simulink model "RCAM_simulation_MIMO"  (R2021b)
settings: Solver=VariableStepAuto  StartTime=0.0  StopTime=TF  FixedStep=0.0001  RelTol=1e-3
values from neighbouring files (symbols this model uses):
  h0 = 1000    [initializeConstantsMIMO.m]
  k = k_gain.K    [initializeConstantsMIMO.m]
  lat0 = convert_coordinates(21, 18, 56.1708)    [initializeConstantsMIMO.m]
  lon0 = convert_coordinates(157, 51, 29.1348)    [initializeConstantsMIMO.m]
  u1max = 25*pi/180    (= 0.436332312999)    [initializeConstantsMIMO.m]
  u1min = -25*pi/180    (= -0.436332312999)    [initializeConstantsMIMO.m]
  u2max = 10*pi/180    (= 0.174532925199)    [initializeConstantsMIMO.m]
  u2min = -25*pi/180    (= -0.436332312999)    [initializeConstantsMIMO.m]
  u3max = 30*pi/180    (= 0.523598775598)    [initializeConstantsMIMO.m]
  u3min = -30*pi/180    (= -0.523598775598)    [initializeConstantsMIMO.m]
  u4max = 1    [initializeConstantsMIMO.m]
  u4min = 0    [initializeConstantsMIMO.m]
  uo = [0 ... (first row only)    [initializeConstantsMIMO.m]
  x0 = [14 ... (first row only)    [initializeConstantsMIMO.m]
undefined symbols (not defined in the file or in its folder): RCAM_model
libraries: aerolibfltsims x2, slpidlib x1
settings Model: PacingRate=3  Creator=khanh  LastModifiedBy=khanh

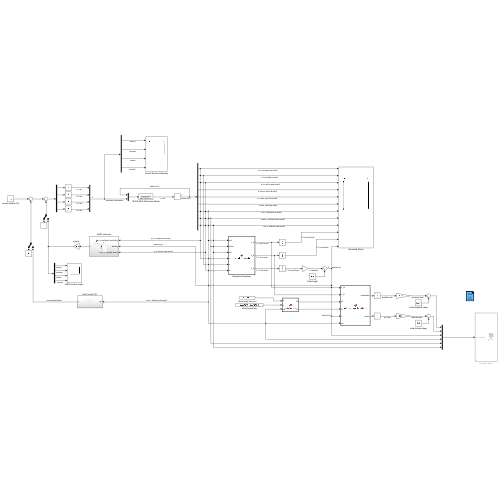
[thumbnail: Simulink's stored preview of the top-level diagram]
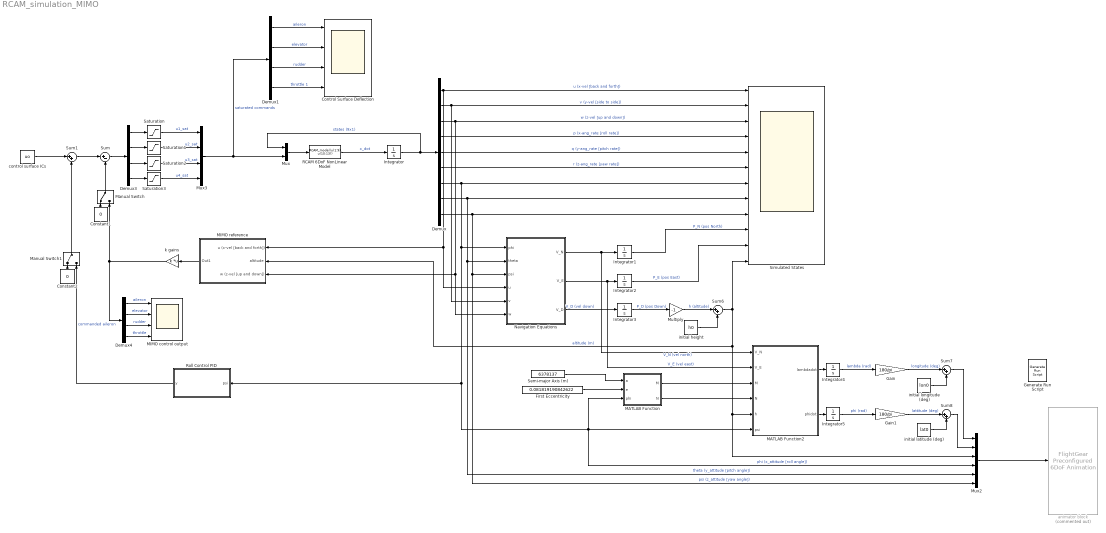
== system RCAM_simulation_MIMO ==
  Constant1 : Constant  Value=0
  Constant2 : Constant  Value=0
  Control Surface Deflection : Scope  NumInputPorts=4
  Demux : Demux  Outputs=9
  Demux1 : Demux
  Demux3 : Demux
  Demux4 : Demux
  First Eccentricity : Constant  Value=0.081819190842622
  Gain : Gain  Gain=180/pi
  Gain1 : Gain  Gain=180/pi
  Generate Run Script : aerolibfltsims/Generate Run Script  Architecture=Win64  dataFlow=Send  GeometryModelName=c172p  AirportId=KSFO  RunwayId=10L  InitialAltitude=7224  InitialHeading=113  OffsetDistance=4.72  OffsetAzimuth=0  InstallScenery=off  DisableShaders=on  OriginAddress=127.0.0.1  DestinationPort=5502  OriginPort=5505  LocalAddress=127.0.0.1  OutputFileName=runfg.bat  FlightGearBaseDirectory=C:\Program Files\FlightGear 2020.3
  Integrator : Integrator  InitialCondition=x0
  Integrator{1..4} (4 alike) : Integrator
  Integrator5 : Integrator  UpperSaturationLimit=pi  LowerSaturationLimit=-pi
  MATLAB Function : MATLAB Function  TreatAsAtomicUnit=on
  MATLAB Function2 : MATLAB Function  TreatAsAtomicUnit=on
  MIMO control output : Scope  NumInputPorts=4
  MIMO reference : Subsystem
  Manual Switch : ManualSwitch
  Manual Switch1 : ManualSwitch
  Multiply : Gain  Gain=-1
  Mux : Mux  Inputs=2
  Mux2 : Mux  Inputs=6
  Mux3 : Mux
  Navigation Equations : MATLAB Function  TreatAsAtomicUnit=on
  RCAM 6DoF NonLinear Model : MATLABFcn  MATLABFcn=RCAM_model(u(1:9), u(10:13))
  Roll Control PID : Subsystem
  Saturation : Saturate  UpperLimit=u1max  LowerLimit=u1min
  Saturation1 : Saturate  UpperLimit=u2max  LowerLimit=u2min
  Saturation2 : Saturate  UpperLimit=u3max  LowerLimit=u3min
  Saturation3 : Saturate  UpperLimit=u4max  LowerLimit=u4min
  Semi-major Axis (m) : Constant  Value=6378137
  Simulated States : Scope  NumInputPorts=12
  Sum : Sum  Inputs=|+-
  Sum{1,6..8} (4 alike) : Sum  Inputs=|++
  animator block : aerolibfltsims/FlightGear Preconfigured 6DoF Animation  Commented=on  xFlightGearVersion=v2019.1  DestinationIpAddress=127.0.0.1  DestinationPort=5502  SampleTime=1/30  packetVersion=24
  control surface ICs : Constant  Value=uo
  initial height : Constant  Value=h0
  initial latitude (deg) : Constant  Value=lat0
  initial longitude (deg) : Constant  Value=lon0
  k gains : Gain  Gain=k  Multiplication=Matrix(K*u)
  wires:
  RCAM 6DoF NonLinear Model/1 -> Integrator/1  "x_dot"
  Mux/1 -> RCAM 6DoF NonLinear Model/1
  Mux3/1 -> Demux1/1, Mux/2  "saturated commands"
  Demux1/1 -> Control Surface Deflection/1  "aileron"
  Demux1/2 -> Control Surface Deflection/2  "elevator"
  Demux1/3 -> Control Surface Deflection/3  "rudder"
  Demux1/4 -> Control Surface Deflection/4  "throttle 1"
  Demux/4 -> Simulated States/4  "p (x-ang_rate [roll rate])"
  Demux/5 -> Simulated States/5  "q (y-ang_rate [pitch rate])"
  Demux/6 -> Simulated States/6  "r (z-ang_rate [yaw rate])"
  Demux/9 -> Mux2/6, Navigation Equations/3(psi), Simulated States/9  "psi (z_attitude [yaw angle])"
  Navigation Equations/3(V_D) -> Integrator3/1  "V_D (vel down)"
  Navigation Equations/2(V_E) -> Integrator2/1, MATLAB Function2/2(V_E)  "V_E (vel east)"
  Navigation Equations/1(V_N) -> MATLAB Function2/1(V_N), Integrator1/1  "V_N (vel north)"
  Integrator1/1 -> Simulated States/10  "P_N (pos North)"
  Integrator2/1 -> Simulated States/11  "P_E (pos East)"
  Integrator3/1 -> Multiply/1  "P_D (pos Down)"
  Semi-major Axis (m)/1 -> MATLAB Function/1(a)
  First Eccentricity/1 -> MATLAB Function/2(e)
  MATLAB Function/2(N) -> MATLAB Function2/4(N)
  MATLAB Function/1(M) -> MATLAB Function2/3(M)
  Demux/7 -> Roll Control PID/1(psi), MATLAB Function2/6(psi), MATLAB Function/3(phi), Mux2/4, Navigation Equations/1(phi), Simulated States/7  "phi (x_attitude [roll angle])"
  Integrator5/1 -> Gain1/1  "phi (rad)"
  Integrator4/1 -> Gain/1  "lambda (rad)"
  Gain/1 -> Sum7/1  "longitude (deg)"
  Multiply/1 -> Sum6/1  "h (altitude)"
  Sum6/1 -> Simulated States/12, MIMO reference/2(altitude), Mux2/3, MATLAB Function2/5(h)  "altitude (m)"
  initial height/1 -> Sum6/2
  MATLAB Function2/1(lambdadot) -> Integrator4/1
  MATLAB Function2/2(phidot) -> Integrator5/1
  Gain1/1 -> Sum8/1  "lattitude (deg)"
  initial longitude (deg)/1 -> Sum7/2
  initial latitude (deg)/1 -> Sum8/2
  Sum7/1 -> Mux2/1
  Sum8/1 -> Mux2/2
  Roll Control PID/1(y) -> Manual Switch1/2  "commanded aileron"
  Saturation3/1 -> Mux3/4  "u4_sat"
  Saturation/1 -> Mux3/1  "u1_sat"
  Saturation1/1 -> Mux3/2  "u2_sat"
  Saturation2/1 -> Mux3/3  "u3_sat"
  Demux3/1 -> Saturation/1
  Demux3/2 -> Saturation1/1
  Demux3/3 -> Saturation2/1
  Demux3/4 -> Saturation3/1
  Demux/3 -> MIMO reference/3(w (z-vel [up and down])), Navigation Equations/6(w), Simulated States/3  "w (z-vel [up and down])"
  Demux/8 -> Mux2/5, Navigation Equations/2(theta), Simulated States/8  "theta (y_attitude [pitch angle])"
  Demux/1 -> Simulated States/1, Navigation Equations/4(u), MIMO reference/1(u (x-vel [back and forth]))  "u (x-vel [back and forth])"
  Demux/2 -> Simulated States/2, Navigation Equations/5(v)  "v (y-vel [side to side])"
  Sum/1 -> Demux3/1
  k gains/1 -> Manual Switch/2, Demux4/1
  Manual Switch/1 -> Sum/2
  Constant1/1 -> Manual Switch/1
  Constant2/1 -> Manual Switch1/1
  Demux4/3 -> MIMO control output/3  "rudder"
  Demux4/4 -> MIMO control output/4  "throttle"
  Demux4/2 -> MIMO control output/2  "elevator"
  Demux4/1 -> MIMO control output/1  "aileron"
  Integrator/1 -> Mux/1, Demux/1  "states (9x1)"
  Mux2/1 -> animator block/1
  Sum1/1 -> Sum/1
  control surface ICs/1 -> Sum1/1
  MIMO reference/1(Out1) -> k gains/1
  Manual Switch1/1 -> Sum1/2

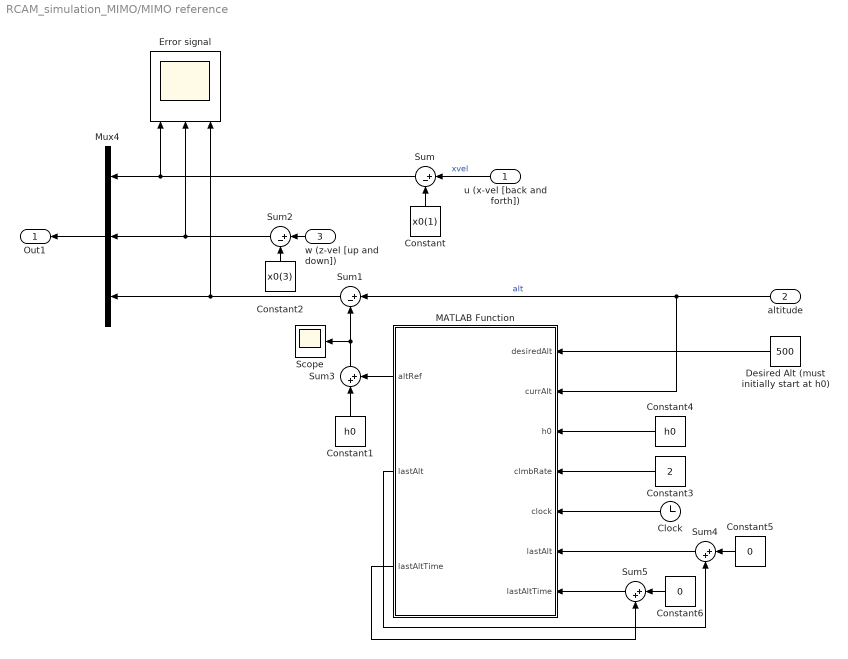
== system RCAM_simulation_MIMO/MIMO reference ==
  u (x-vel [back and forth]) : Inport
  altitude : Inport  Port=2
  w (z-vel [up and down]) : Inport  Port=3
  Clock : Clock
  Constant : Constant  Value=x0(1)
  Constant1 : Constant  Value=h0
  Constant2 : Constant  Value=x0(3)
  Constant3 : Constant  Value=2
  Constant4 : Constant  Value=h0
  Constant5 : Constant  Value=0
  Constant6 : Constant  Value=0
  Desired Alt (must initially start at h0) : Constant  Value=500
  Error signal : Scope  NumInputPorts=3
  MATLAB Function : MATLAB Function  TreatAsAtomicUnit=on
  Mux4 : Mux  Inputs=3
  Scope : Scope
  Sum : Sum  Inputs=|+-
  Sum1 : Sum  Inputs=|+-
  Sum2 : Sum  Inputs=|+-
  Sum3 : Sum  Inputs=|++
  Sum4 : Sum  Inputs=|++
  Sum5 : Sum  Inputs=|++
  Out1 : Outport
  wires:
  Mux4/1 -> Out1/1
  u (x-vel [back and forth])/1 -> Sum/1  "xvel"
  Constant/1 -> Sum/2
  Sum1/1 -> Mux4/3, Error signal/3
  w (z-vel [up and down])/1 -> Sum2/1
  Sum2/1 -> Mux4/2, Error signal/2
  Constant2/1 -> Sum2/2
  Sum/1 -> Mux4/1, Error signal/1
  altitude/1 -> Sum1/1, MATLAB Function/2(currAlt)  "alt"
  MATLAB Function/1(altRef) -> Sum3/2
  Desired Alt (must initially start at h0)/1 -> MATLAB Function/1(desiredAlt)
  Constant4/1 -> MATLAB Function/3(h0)
  Sum3/1 -> Sum1/2, Scope/1
  Constant1/1 -> Sum3/1
  Constant3/1 -> MATLAB Function/4(clmbRate)
  Clock/1 -> MATLAB Function/5(clock)
  MATLAB Function/2(lastAlt) -> Sum4/2
  Sum4/1 -> MATLAB Function/6("lastAlt ")
  Constant5/1 -> Sum4/1
  Constant6/1 -> Sum5/1
  Sum5/1 -> MATLAB Function/7("lastAltTime ")
  MATLAB Function/3(lastAltTime) -> Sum5/2

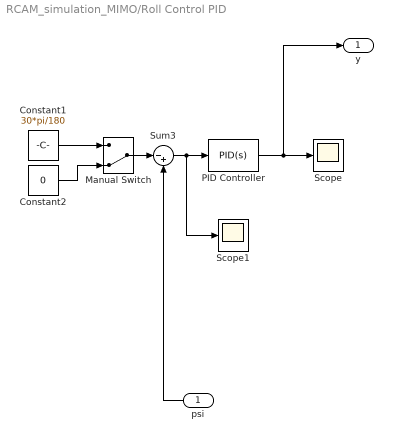
== system RCAM_simulation_MIMO/Roll Control PID ==
  psi : Inport
  Constant1 : Constant  Value=30*pi/180
  Constant2 : Constant  Value=0
  Manual Switch : ManualSwitch  CurrentSetting=0
  PID Controller : slpidlib/PID Controller  Controller=PID  Form=Parallel  TimeDomain=Continuous-time  UseExternalTs=off  SampleTime=-1  IntegratorMethod=Forward Euler  FilterMethod=Forward Euler  ControllerParametersSource=internal  P=0.0579119513751783  I=0.00415622231260998  D=-0.0770290239764599  UseFilter=on  N=0.0600432083940748  TunerSelectOption=Transfer Function Based (PID Tuner App)  InitialConditionSource=internal  InitialConditionForIntegrator=0  InitialConditionForFilter=0  DifferentiatorICPrevScaledInput=0  ExternalReset=none  TrackingMode=off  Kt=1  LimitOutput=on  SatLimitsSource=internal  UpperSaturationLimit=u1max  LowerSaturationLimit=u1min  LinearizeAsGain=on  AntiWindupMode=none  Kb=1  POutMin=[]  POutMax=[]  IOutMin=[]  IOutMax=[]  DOutMin=[]  DOutMax=[]  NOutMin=[]  NOutMax=[]  SumOutMin=[]  SumOutMax=[]  SaturationOutMin=[]  SaturationOutMax=[]  PParamMin=[]  PParamMax=[]  IParamMin=[]  IParamMax=[]  DParamMin=[]  DParamMax=[]  NParamMin=[]  NParamMax=[]  KbParamMin=[]  KbParamMax=[]  KtParamMin=[]  KtParamMax=[]  KbOutMin=[]  KbOutMax=[]  KtOutMin=[]  KtOutMax=[]  IntegratorOutMin=[]  IntegratorOutMax=[]  FilterOutMin=[]  FilterOutMax=[]  SumI1OutMin=[]  SumI1OutMax=[]  SumI2OutMin=[]  SumI2OutMax=[]  SumI3OutMin=[]  SumI3OutMax=[]  SumI4OutMin=[]  SumI4OutMax=[]  SumDOutMin=[]  SumDOutMax=[]  DifferentiatorOutMin=[]  DifferentiatorOutMax=[]  FilterDiffOutCoefMin=[]  FilterDiffOutCoefMax=[]  ReciprocalOutMin=[]  ReciprocalOutMax=[]  SumDenOutMin=[]  SumDenOutMax=[]  SumNumOutMin=[]  SumNumOutMax=[]  DivideOutMin=[]  DivideOutMax=[]  UdiffTsProdOutMin=[]  UdiffTsProdOutMax=[]  NTsProdOutMin=[]  NTsProdOutMax=[]  UintegralTsProdOutMin=[]  UintegralTsProdOutMax=[]  UngainTsProdOutMin=[]  UngainTsProdOutMax=[]  IntegratorContinuousStateAttributes=''  IntegratorStateMustResolveToSignalObject=off  IntegratorRTWStateStorageClass=Auto  FilterContinuousStateAttributes=''  FilterStateMustResolveToSignalObject=off  FilterRTWStateStorageClass=Auto  ParallelPVariant=InternalParameters  IdealPVariant=Disabled  IVariant=InternalParameters  DVariant=InternalParameters  IntegratorVariant=Continuous  SatVariant=Enabled  AWVariant=Passthrough  PCopyVariant=Disabled  TRVariant=Disabled  FdbkBlocksVariant=Forward  IdealPFdbkVariant=Disabled  SatFdbkVariant=Disabled  DerivativeFilterVariant=ContFilter  NVariant=InternalParameters  NCopyVariant=Disabled  FilterICVariant=InternalICsFilter  IntegratorICVariant=InternalICs  ExternalResetVariant=Disabled  TRSumVariant=Passthrough  SumFdbkVariant=Disabled  SumVariant=Sum_PID  TsampFilterVariant=InternalTs  TsampNgainVariant=Passthrough  TsampIntegralVariant=Passthrough  ExternalSaturationOutDataTypeStr=Inherit: Same as second input
  Scope : Scope
  Scope1 : Scope
  Sum3 : Sum  Inputs=|-+
  y : Outport
  wires:
  Constant1/1 -> Manual Switch/1
  Sum3/1 -> Scope1/1, PID Controller/1
  Manual Switch/1 -> Sum3/1
  Constant2/1 -> Manual Switch/2
  psi/1 -> Sum3/2
  PID Controller/1 -> y/1, Scope/1

== matlab function RCAM_simulation_MIMO/MATLAB Function ==
  data: a input; M output; e input; phi input; N output
function [M, N] = calculate_mn (a, e, phi)

M = a*(1-e^2)/(1-(e^2)*sin(phi)^2)^1.5;

N = a/(1-(e^2)*sin(phi)^2)^0.5;

end

== matlab function RCAM_simulation_MIMO/Navigation Equations ==
  data: phi input; theta input; psi input; u input; V_N output; v input; w input; V_E output; V_D output
function [V_N, V_E, V_D] = navigation_equation(phi, theta, psi, u, v, w)

x7 = phi;
x8 = theta;
x9 = psi;
x1 = u;
x2 = v;
x3 = w;

V_b = [x1; x2; x3];

%navigation equations
C1v = [cos(x9) sin(x9) 0; -sin(x9) cos(x9) 0; 0 0 1];

C21 = [cos(x8) 0 -sin(x8); 0 1 0; sin(x8) 0 cos(x8)];

Cb2 = [1 0 0; 0 cos(x7) sin(x7); 0 -sin(x7) cos(x7)];

Cvb = Cb2*C21*C1v;
Cvb = Cvb';

vel_vector = Cvb*V_b;

V_N = vel_vector(1);
V_E = vel_vector(2);
V_D = vel_vector(3);

end

== matlab function RCAM_simulation_MIMO/MIMO reference/MATLAB Function ==
  data: desiredAlt input; altRef output; currAlt input; h0 input; clmbRate input; clock input; lastAlt input; lastAlt output; lastAltTime input; lastAltTime output
function [altRef, lastAlt, lastAltTime] = altitudeControl(desiredAlt, currAlt, h0, clmbRate, clock, lastAlt, lastAltTime)
    
    %if currAlt is above or below desired alt, initiate climb/descent
    %if currAlt is within 10% of desired alt, initiate alt lock

    tol = 0.1*abs(desiredAlt-currAlt);
    rampSignal = (clock)*clmbRate-(lastAltTime*clmbRate+h0-lastAlt);

    if tol < 10 %setting absolute tolerance, this number will be higher as climb rate increases
        tol = clmbRate*3;
    end
   
    if currAlt < desiredAlt - tol
        rampSignal = (clock)*clmbRate-((lastAltTime*clmbRate+h0)-lastAlt);
        altRef = rampSignal;

    elseif currAlt > desiredAlt + tol
        rampSignal = -1*(clock)*clmbRate+(lastAlt-(lastAltTime*-1*clmbRate+h0));
        altRef = rampSignal;

    else
        altRef = desiredAlt-h0;
        lastAlt = currAlt;
        lastAltTime = clock;
    end
end

== matlab function RCAM_simulation_MIMO/MATLAB Function2 ==
  data: lambdadot output; V_N input; V_E input; phidot output; M input; N input; h input; psi input
function [lambdadot, phidot] = calculate_phi_lambdadot(V_N, V_E, M, N, h, psi)

lambdadot = V_E/(N+h)*cos(psi);
phidot = V_N/(M+h);


end
